simulink model "SpringiLQR2discrete"  (R2021a)
settings: Solver=FixedStepAuto  StartTime=0.0  StopTime=100  FixedStep=0.01  MaxStep=0.01  RelTol=1e-3
values from neighbouring files (symbols this model uses):
  b = 3    [SringiLQR.m]    (also in SringiLQR2.m; SringiLQR2discrete.m; SringiLQR3discrete.m = 0.01; test123.m = 0.01)
  k = 1    [SringiLQR.m]    (also in SringiLQR2.m; SringiLQR2discrete.m; SringiLQR3discrete.m = 0; extmodel.m = 10)
  mass = 1    [SringiLQR.m]    (also in SringiLQR2.m; SringiLQR2discrete.m; SringiLQR3discrete.m; test123.m)
  Q = [1 0 0; 0 1 0; 0 0 10]    [LQR.m]    (also in NonlinearVehicleLQR.m = eye(3)*10; NonlinearVehicleiLQR.m = eye(3)*10; SringiLQR.m = [1 0; 0 1]*1; SringiLQR2.m = [1 0; 0 1]*1)
  Qf = eye(3)    [LQR.m]    (also in NonlinearVehicleLQR.m; NonlinearVehicleiLQR.m; SringiLQR.m = [1 0; 0 1]; SringiLQR2.m = [1 0; 0 1])
  R = eye(2)*10^-4    [LQR.m]    (also in NonlinearVehicleLQR.m = eye(2)*10^-2; NonlinearVehicleiLQR.m = eye(2)*10^-2; SringiLQR.m = eye(1)*1e-2; SringiLQR2.m = eye(1)*1e-2)
libraries: simulink x1, pid_lib x1
settings Model: Creator=iris  LastModifiedBy=iris
settings SolverCC: AlgebraicLoopSolver=TrustRegion

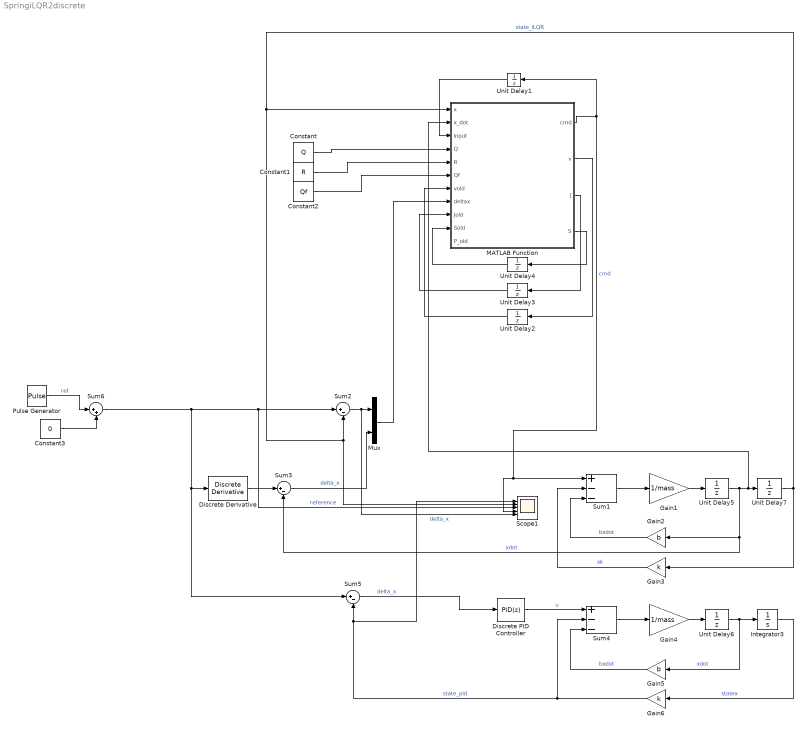
== system SpringiLQR2discrete ==
  Constant : Constant  Value=Q
  Constant1 : Constant  Value=R
  Constant2 : Constant  Value=Qf
  Constant3 : Constant  Value=0
  Discrete Derivative : simulink/Discrete/Discrete Derivative  gainval=1.0  ICPrevScaledInput=0.0  OutMin=[]  OutMax=[]  OutDataType=fixdt(1, 16)  OutScaling=2^-10  DoSatur=off
  Discrete PID Controller : pid_lib/PID Controller  Controller=PID  Form=Parallel  TimeDomain=Discrete-time  UseExternalTs=off  SampleTime=-1  IntegratorMethod=Forward Euler  FilterMethod=Forward Euler  ControllerParametersSource=internal  P=8  I=4  D=3  UseFilter=on  N=100  TunerSelectOption=Transfer Function Based (PID Tuner App)  InitialConditionSource=internal  InitialConditionForIntegrator=0  InitialConditionForFilter=0  DifferentiatorICPrevScaledInput=0  ExternalReset=none  TrackingMode=off  Kt=1  LimitOutput=off  SatLimitsSource=internal  UpperSaturationLimit=inf  LowerSaturationLimit=-inf  LinearizeAsGain=off  AntiWindupMode=none  Kb=1  POutMin=[]  POutMax=[]  IOutMin=[]  IOutMax=[]  DOutMin=[]  DOutMax=[]  NOutMin=[]  NOutMax=[]  SumOutMin=[]  SumOutMax=[]  SaturationOutMin=[]  SaturationOutMax=[]  PParamMin=[]  PParamMax=[]  IParamMin=[]  IParamMax=[]  DParamMin=[]  DParamMax=[]  NParamMin=[]  NParamMax=[]  KbParamMin=[]  KbParamMax=[]  KtParamMin=[]  KtParamMax=[]  KbOutMin=[]  KbOutMax=[]  KtOutMin=[]  KtOutMax=[]  IntegratorOutMin=[]  IntegratorOutMax=[]  FilterOutMin=[]  FilterOutMax=[]  SumI1OutMin=[]  SumI1OutMax=[]  SumI2OutMin=[]  SumI2OutMax=[]  SumI3OutMin=[]  SumI3OutMax=[]  SumI4OutMin=[]  SumI4OutMax=[]  SumDOutMin=[]  SumDOutMax=[]  DifferentiatorOutMin=[]  DifferentiatorOutMax=[]  FilterDiffOutCoefMin=[]  FilterDiffOutCoefMax=[]  ReciprocalOutMin=[]  ReciprocalOutMax=[]  SumDenOutMin=[]  SumDenOutMax=[]  SumNumOutMin=[]  SumNumOutMax=[]  DivideOutMin=[]  DivideOutMax=[]  UdiffTsProdOutMin=[]  UdiffTsProdOutMax=[]  NTsProdOutMin=[]  NTsProdOutMax=[]  UintegralTsProdOutMin=[]  UintegralTsProdOutMax=[]  UngainTsProdOutMin=[]  UngainTsProdOutMax=[]  IntegratorContinuousStateAttributes=''  IntegratorStateMustResolveToSignalObject=off  IntegratorRTWStateStorageClass=Auto  FilterContinuousStateAttributes=''  FilterStateMustResolveToSignalObject=off  FilterRTWStateStorageClass=Auto  ParallelPVariant=InternalParameters  IdealPVariant=Disabled  IVariant=InternalParameters  DVariant=InternalParameters  IntegratorVariant=Discrete  SatVariant=Disabled  AWVariant=Passthrough  PCopyVariant=Disabled  TRVariant=Disabled  FdbkBlocksVariant=Forward  IdealPFdbkVariant=Disabled  SatFdbkVariant=Disabled  DerivativeFilterVariant=ForwardEulerFilter  NVariant=InternalParameters  NCopyVariant=Disabled  FilterICVariant=InternalICsFilter  IntegratorICVariant=InternalICs  ExternalResetVariant=Disabled  TRSumVariant=Passthrough  SumFdbkVariant=Disabled  SumVariant=Sum_PID  TsampFilterVariant=InternalTs  TsampNgainVariant=Passthrough  TsampIntegralVariant=Passthrough  ExternalSaturationOutDataTypeStr=Inherit: Same as second input
  Gain1 : Gain  Gain=1/mass
  Gain2 : Gain  Gain=b
  Gain3 : Gain  Gain=k
  Gain4 : Gain  Gain=1/mass
  Gain5 : Gain  Gain=b
  Gain6 : Gain  Gain=k
  Integrator3 : Integrator
  MATLAB Function : MATLAB Function  TreatAsAtomicUnit=on
  Mux : Mux  Inputs=2
  Pulse Generator : DiscretePulseGenerator  PulseType=Time based  Period=20  PulseWidth=50
  Scope1 : Scope  NumInputPorts=5
  Sum1 : Sum  Inputs=+--
  Sum2 : Sum  Inputs=|+-
  Sum3 : Sum  Inputs=|+-
  Sum4 : Sum  Inputs=+--
  Sum5 : Sum  Inputs=|+-
  Sum6 : Sum  Inputs=|++
  Unit Delay{1,5..7} (4 alike) : UnitDelay  SampleTime=-1  HasFrameUpgradeWarning=on
  Unit Delay2 : UnitDelay  InitialCondition=zeros(2,1)  SampleTime=-1  HasFrameUpgradeWarning=on
  Unit Delay3 : UnitDelay  InitialCondition=10000  SampleTime=-1  HasFrameUpgradeWarning=on
  Unit Delay4 : UnitDelay  InitialCondition=Qf  SampleTime=-1  HasFrameUpgradeWarning=on
  wires:
  Gain1/1 -> Unit Delay5/1
  Sum1/1 -> Gain1/1
  Unit Delay5/1 -> Sum3/2, Gain2/1, Unit Delay7/1, MATLAB Function/2(x_dot)  "xdot"
  Gain3/1 -> Sum1/2  "xk"
  Gain2/1 -> Sum1/3  "bxdot"
  Pulse Generator/1 -> Sum6/1  "ref"
  Sum2/1 -> Mux/1, Scope1/5  "delta_x"
  Unit Delay7/1 -> Gain3/1, Scope1/2, Sum2/2, MATLAB Function/1(x)  "state_iLQR"
  MATLAB Function/3(J) -> Unit Delay3/1
  MATLAB Function/2(v) -> Unit Delay2/1
  Constant/1 -> MATLAB Function/4(Q)
  Constant2/1 -> MATLAB Function/6(Qf)
  Constant1/1 -> MATLAB Function/5(R)
  MATLAB Function/1(cmd) -> Scope1/4, Sum1/1, Unit Delay1/1  "cmd"
  Unit Delay2/1 -> MATLAB Function/7(vold)
  Discrete Derivative/1 -> Sum3/1
  Sum3/1 -> Mux/2  "delta_x"
  Mux/1 -> MATLAB Function/8(deltax)
  Integrator3/1 -> Gain6/1  "statex"
  Gain5/1 -> Sum4/3  "bxdot"
  Gain6/1 -> Scope1/1, Sum5/2, Sum4/2  "state_pid"
  Unit Delay6/1 -> Integrator3/1, Gain5/1  "xdot"
  Sum4/1 -> Gain4/1
  Gain4/1 -> Unit Delay6/1
  Discrete PID Controller/1 -> Sum4/1  "u"
  Sum5/1 -> Discrete PID Controller/1  "delta_x"
  Constant3/1 -> Sum6/2
  Sum6/1 -> Scope1/3, Sum2/1, Discrete Derivative/1, Sum5/1  "reference"
  Unit Delay1/1 -> MATLAB Function/3(input)
  Unit Delay3/1 -> MATLAB Function/9(Jold)
  MATLAB Function/4(S) -> Unit Delay4/1
  Unit Delay4/1 -> MATLAB Function/10(Sold)

== matlab function SpringiLQR2discrete/MATLAB Function ==
  data: x input; x_dot input; input input; Q input; R input; Qf input; vold input; deltax input; cmd output; Jold input; Sold input; v output; J output; S output; P_old input
function [cmd, v, J, S]= fcn(x,x_dot, input, Q, R, Qf, vold, deltax, Jold, Sold,P_old)

% r = 0.02;
% B = 0.185;
% dt = 0.01;
k = 1;
b = 3;
mass = 1;


toll = 3*10^-5;

A = [0 1;...
     -k/mass -b/mass];
B = [0;1];
state = [x,x_dot];
J = state*Qf*state'+state*Q*state'+input*R*input';
cmd = zeros(1,1);

if abs(Jold-J)/Jold > toll
    K  = (B'*Sold*B+R)\B'*Sold*A;
    Kv = (B'*Sold*B+R)\B';
    Ku = (B'*Sold*B+R)\R;
    S  = A'*Sold*(A-B*K)+Q;
    v  = (A-B*K)'*vold+Q*state'-K'*R*input';
    deltau = -K*deltax-Kv*v-Ku*input';

    cmd  = input' + deltau;
%   Alternative from https://people.eecs.berkeley.edu/~pabbeel/cs287-fa12/slides/LQR.pdf
%     K_iter = -1*(R+B'*P_old*B)\B'*P_old*A;
%     P_iter = Q + K_iter'*R*K_iter + (A+B*K_iter)'*P_old*(A+B*K_iter);
%     f = -1*(R+B'*P_old*B)\B'*(P_iter
%     cmd = K_iter*(deltax+state');  % -k*reference
else
    S  = Sold;
    v  = vold;
    cmd  = input';
% Alternative
    P_iter = P_old;


end
